simulink library "Lib_EMTAT"  (R2023b)
settings: Solver=VariableStepAuto  StartTime=0.0  StopTime=10.0  RelTol=1e-3
undefined symbols (not defined in the file): MWS
libraries: simulink x34
(part 2 of 4)

== system Lib_EMTAT/Components/Power Flow/Cable ==
  note: Memory block used to break algebraic loop.
  "V_1, V" : Inport
  "I, A" : Inport  Port=2
  Fail? : Inport  Port=3
  "I(t-1), A" : Inport  Port=4
  Bus Creator : BusCreator  Inputs=7
  Constant : Constant  Value=R
  Divide{,1..3} (4 alike) : Product  Inputs=**
  Failure Determination : Subsystem
  Fix Zero Voltage Problem : Subsystem
  Open Circuit Failure - Current : Subsystem
  Open Circuit Failure - Voltage : Subsystem
  Square : Math  Operator=square
  Sum : Sum  Inputs=|-+
  "V_2, V" : Outport
  Outputs : Outport  Port=2
  "Ploss, W" : Outport  Port=3
  "I, A " : Outport  Port=4
  "I(t), A" : Outport  Port=5
  wires:
  [OCFail] -> Open Circuit Failure - Voltage/1(Failed?)
  Fix Zero Voltage Problem/1(Vout) -> Open Circuit Failure - Voltage/2(Vout)
  [OCFail] -> Open Circuit Failure - Current/1(Failed?)
  Open Circuit Failure - Current/1("Iin/Iout ") -> "I, A "/1, [Iin], Divide2/2, Divide3/1, Square/1
  "I, A"/1 -> "I(t), A"/1, Open Circuit Failure - Current/2(Iin/Iout)
  Fail?/1 -> Failure Determination/1(Fail?)
  Failure Determination/1(OCFail) -> [OCFail]
  "I(t-1), A"/1 -> Divide/1
  Divide/1 -> Sum/1
  "V_1, V"/1 -> Divide2/1, Sum/2, Fix Zero Voltage Problem/2(Vin), [Vin]
  Sum/1 -> Fix Zero Voltage Problem/1("Vout "), Divide3/2
  [Iin] -> Bus Creator/3  "I; A"
  [Vout] -> Bus Creator/5  "V_2; V"
  [Vin] -> Bus Creator/4  "V_1; V"
  Bus Creator/1 -> Outputs/1
  [R] -> Bus Creator/6  "R; ohm"
  Constant/1 -> Divide1/2, [R], Divide/2
  Square/1 -> Divide1/1
  Divide1/1 -> [Ploss], "Ploss, W"/1
  [Pin] -> Bus Creator/2  "P_1; W"
  [Pout] -> Bus Creator/1  "P_2; W"
  Divide2/1 -> [Pin]
  Divide3/1 -> [Pout]
  [Ploss] -> Bus Creator/7  "Ploss; W"
  Open Circuit Failure - Voltage/1("Vout ") -> "V_2, V"/1, [Vout]

== system Lib_EMTAT/Components/Power Flow/Current Distribution ==
  "I, A" : Inport
  "Idmd, A" : Inport  Port=2
  MATLAB Function : MATLAB Function  TreatAsAtomicUnit=on
  "Isplit, A" : Outport
  wires:
  "Idmd, A"/1 -> MATLAB Function/2(Idmd)
  MATLAB Function/1(Isplit) -> "Isplit, A"/1
  "I, A"/1 -> MATLAB Function/1(I)

== system Lib_EMTAT/Components/Power Flow/Current Junction ==
  I : Inport
  MATLAB Function : MATLAB Function  TreatAsAtomicUnit=on
  Isum : Outport
  wires:
  I/1 -> MATLAB Function/1(u)
  MATLAB Function/1(y) -> Isum/1

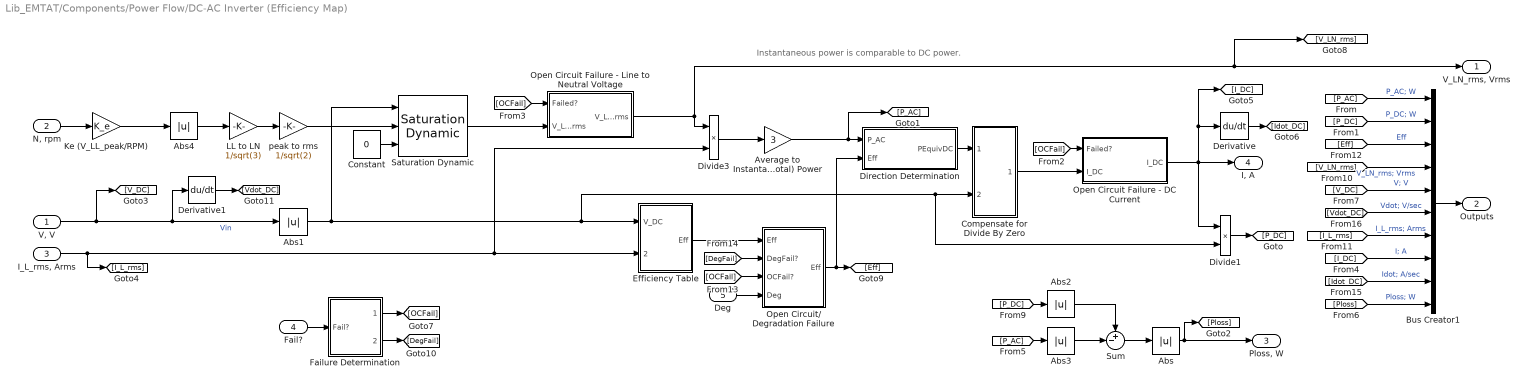
== system Lib_EMTAT/Components/Power Flow/DC-AC Inverter (Efficiency Map) ==
  note: Instantaneous power is comparable to DC power.
  "V, V" : Inport
  "N, rpm" : Inport  Port=2
  "I_L_rms, Arms" : Inport  Port=3
  Fail? : Inport  Port=4
  Deg : Inport  Port=5
  Abs{,1..4} (5 alike) : Abs  SaturateOnIntegerOverflow=off
  Average to Instantaneous (Total) Power : Gain  Gain=3
  Bus Creator1 : BusCreator  Inputs=10
  Compensate for Divide By Zero : Subsystem
  Constant : Constant  Value=0
  Derivative : Derivative
  Derivative1 : Derivative
  Direction Determination : Subsystem
  Divide1 : Product  Inputs=**
  Divide3 : Product  Inputs=**
  Efficiency Table : Subsystem
  Failure Determination : Subsystem
  Ke (V_LL_peak/RPM) : Gain  Gain=K_e
  LL to LN : Gain  Gain=1/sqrt(3)
  Open Circuit Failure - DC Current : Subsystem
  Open Circuit Failure - Line to Neutral Voltage : Subsystem
  Open Circuit/ Degradation Failure : Subsystem
  Saturation Dynamic : simulink/Discontinuities/Saturation Dynamic  OutMin=[]  OutMax=[]  OutDataTypeStr=Inherit: Same as second input  OutDataType=fixdt(1, 16)  OutScaling=2^-10  DoSatur=off
  Sum : Sum  Inputs=+-|
  peak to rms : Gain  Gain=1/sqrt(2)
  "V_LN_rms, Vrms" : Outport
  Outputs : Outport  Port=2
  "Ploss, W" : Outport  Port=3
  "I, A" : Outport  Port=4
  wires:
  peak to rms/1 -> Saturation Dynamic/2
  Constant/1 -> Saturation Dynamic/3
  Divide3/1 -> Average to Instantaneous (Total) Power/1
  Abs4/1 -> LL to LN/1
  Abs1/1 -> Efficiency Table/1(V_DC), Compensate for Divide By Zero/2(V_DC), Divide1/2, Saturation Dynamic/1
  Divide1/1 -> [P_DC]
  Direction Determination/1(PEquivDC) -> Compensate for Divide By Zero/1(PEquivDC)
  Bus Creator1/1 -> Outputs/1
  [P_AC] -> Bus Creator1/1  "P_AC; W"
  [P_DC] -> Bus Creator1/2  "P_DC; W"
  "N, rpm"/1 -> Ke (V_LL_peak/RPM)/1
  Open Circuit/ Degradation Failure/1("Eff ") -> [Eff], Direction Determination/2(Eff)
  Open Circuit Failure - DC Current/1("I_DC ") -> Divide1/1, "I, A"/1, Derivative/1, [I_DC]
  Average to Instantaneous (Total) Power/1 -> Direction Determination/1(P_AC), [P_AC]
  "V, V"/1 -> Derivative1/1, Abs1/1, [V_DC]  "Vin"
  Ke (V_LL_peak/RPM)/1 -> Abs4/1
  "I_L_rms, Arms"/1 -> Efficiency Table/2(I_L_rms), Divide3/2, [I_L_rms]
  [V_LN_rms] -> Bus Creator1/4  "V_LN_rms; Vrms"
  [V_DC] -> Bus Creator1/5  "V; V"
  [I_DC] -> Bus Creator1/8  "I; A"
  [Ploss] -> Bus Creator1/10  "Ploss; W"
  [I_L_rms] -> Bus Creator1/7  "I_L_rms; Arms"
  [Eff] -> Bus Creator1/3  "Eff"
  LL to LN/1 -> peak to rms/1
  Compensate for Divide By Zero/1(I_DC) -> Open Circuit Failure - DC Current/2(I_DC)
  [OCFail] -> Open Circuit Failure - DC Current/1(Failed?)
  Saturation Dynamic/1 -> Open Circuit Failure - Line to Neutral Voltage/2(V_LN_rms)
  [OCFail] -> Open Circuit Failure - Line to Neutral Voltage/1(Failed?)
  Open Circuit Failure - Line to Neutral Voltage/1("V_LN_rms ") -> [V_LN_rms], "V_LN_rms, Vrms"/1, Divide3/1
  Efficiency Table/1(Eff) -> Open Circuit/ Degradation Failure/1(Eff)
  Failure Determination/2(DegFail) -> [DegFail]
  Failure Determination/1(OCFail) -> [OCFail]
  Fail?/1 -> Failure Determination/1(Fail?)
  Deg/1 -> Open Circuit/ Degradation Failure/4(Deg)
  [OCFail] -> Open Circuit/ Degradation Failure/3(OCFail?)
  [DegFail] -> Open Circuit/ Degradation Failure/2(DegFail?)
  Derivative/1 -> [Idot_DC]
  Derivative1/1 -> [Vdot_DC]
  [Idot_DC] -> Bus Creator1/9  "Idot; A/sec"
  [Vdot_DC] -> Bus Creator1/6  "Vdot; V/sec"
  Sum/1 -> Abs/1
  [P_DC] -> Abs2/1
  Abs3/1 -> Sum/2
  [P_AC] -> Abs3/1
  Abs2/1 -> Sum/1
  Abs/1 -> [Ploss], "Ploss, W"/1

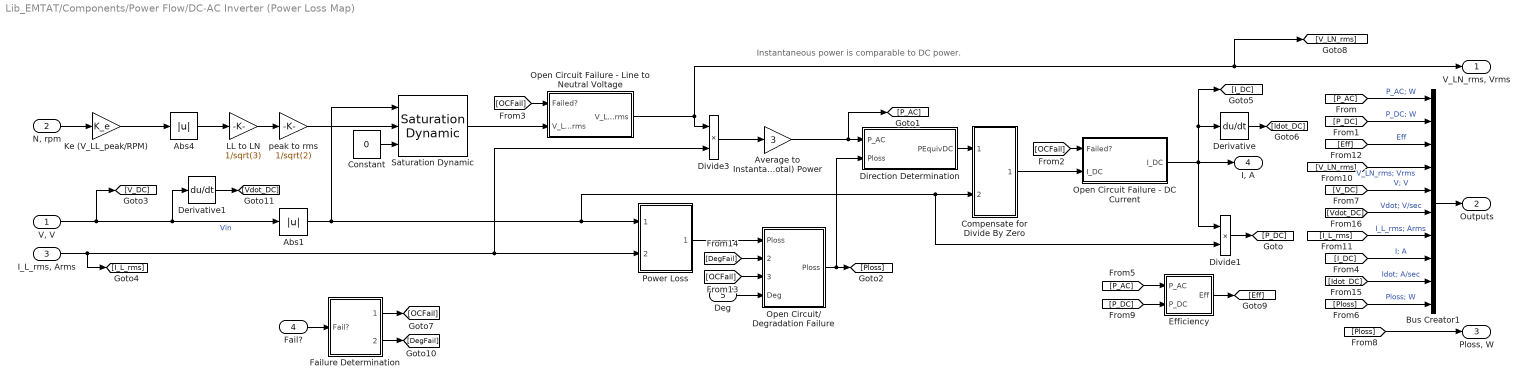
== system Lib_EMTAT/Components/Power Flow/DC-AC Inverter (Power Loss Map) ==
  note: Instantaneous power is comparable to DC power.
  "V, V" : Inport
  "N, rpm" : Inport  Port=2
  "I_L_rms, Arms" : Inport  Port=3
  Fail? : Inport  Port=4
  Deg : Inport  Port=5
  Abs1 : Abs  SaturateOnIntegerOverflow=off
  Abs4 : Abs  SaturateOnIntegerOverflow=off
  Average to Instantaneous (Total) Power : Gain  Gain=3
  Bus Creator1 : BusCreator  Inputs=10
  Compensate for Divide By Zero : Subsystem
  Constant : Constant  Value=0
  Derivative : Derivative
  Derivative1 : Derivative
  Direction Determination : Subsystem
  Divide1 : Product  Inputs=**
  Divide3 : Product  Inputs=**
  Efficiency : Subsystem
  Failure Determination : Subsystem
  Ke (V_LL_peak/RPM) : Gain  Gain=K_e
  LL to LN : Gain  Gain=1/sqrt(3)
  Open Circuit Failure - DC Current : Subsystem
  Open Circuit Failure - Line to Neutral Voltage : Subsystem
  Open Circuit/ Degradation Failure : Subsystem
  Power Loss : Subsystem
  Saturation Dynamic : simulink/Discontinuities/Saturation Dynamic  OutMin=[]  OutMax=[]  OutDataTypeStr=Inherit: Same as second input  OutDataType=fixdt(1, 16)  OutScaling=2^-10  DoSatur=off
  peak to rms : Gain  Gain=1/sqrt(2)
  "V_LN_rms, Vrms" : Outport
  Outputs : Outport  Port=2
  "Ploss, W" : Outport  Port=3
  "I, A" : Outport  Port=4
  wires:
  [Vdot_DC] -> Bus Creator1/6  "Vdot; V/sec"
  [Idot_DC] -> Bus Creator1/9  "Idot; A/sec"
  Derivative1/1 -> [Vdot_DC]
  Derivative/1 -> [Idot_DC]
  [DegFail] -> Open Circuit/ Degradation Failure/2(DegFail?)
  [OCFail] -> Open Circuit/ Degradation Failure/3(OCFail?)
  Deg/1 -> Open Circuit/ Degradation Failure/4(Deg)
  Fail?/1 -> Failure Determination/1(Fail?)
  Failure Determination/1(OCFail) -> [OCFail]
  Failure Determination/2(DegFail) -> [DegFail]
  Power Loss/1(Ploss) -> Open Circuit/ Degradation Failure/1(Ploss)
  Open Circuit Failure - Line to Neutral Voltage/1("V_LN_rms ") -> Divide3/1, "V_LN_rms, Vrms"/1, [V_LN_rms]
  [OCFail] -> Open Circuit Failure - Line to Neutral Voltage/1(Failed?)
  Saturation Dynamic/1 -> Open Circuit Failure - Line to Neutral Voltage/2(V_LN_rms)
  [OCFail] -> Open Circuit Failure - DC Current/1(Failed?)
  Compensate for Divide By Zero/1(I_DC) -> Open Circuit Failure - DC Current/2(I_DC)
  LL to LN/1 -> peak to rms/1
  [Eff] -> Bus Creator1/3  "Eff"
  Efficiency/1(Eff) -> [Eff]
  [P_AC] -> Efficiency/1(P_AC)
  [P_DC] -> Efficiency/2(P_DC)
  [I_L_rms] -> Bus Creator1/7  "I_L_rms; Arms"
  [Ploss] -> Bus Creator1/10  "Ploss; W"
  [I_DC] -> Bus Creator1/8  "I; A"
  [V_DC] -> Bus Creator1/5  "V; V"
  [V_LN_rms] -> Bus Creator1/4  "V_LN_rms; Vrms"
  "I_L_rms, Arms"/1 -> [I_L_rms], Divide3/2, Power Loss/2(I_L_rms)
  [Ploss] -> "Ploss, W"/1
  Ke (V_LL_peak/RPM)/1 -> Abs4/1
  "V, V"/1 -> [V_DC], Abs1/1, Derivative1/1  "Vin"
  Average to Instantaneous (Total) Power/1 -> [P_AC], Direction Determination/1(P_AC)
  Open Circuit Failure - DC Current/1("I_DC ") -> [I_DC], Derivative/1, "I, A"/1, Divide1/1
  Open Circuit/ Degradation Failure/1("Ploss ") -> [Ploss], Direction Determination/2(Ploss)
  "N, rpm"/1 -> Ke (V_LL_peak/RPM)/1
  [P_DC] -> Bus Creator1/2  "P_DC; W"
  [P_AC] -> Bus Creator1/1  "P_AC; W"
  Bus Creator1/1 -> Outputs/1
  Direction Determination/1(PEquivDC) -> Compensate for Divide By Zero/1(PEquivDC)
  Divide1/1 -> [P_DC]
  Abs1/1 -> Saturation Dynamic/1, Divide1/2, Compensate for Divide By Zero/2(V_DC), Power Loss/1(V_DC)
  Abs4/1 -> LL to LN/1
  Divide3/1 -> Average to Instantaneous (Total) Power/1
  Constant/1 -> Saturation Dynamic/3
  peak to rms/1 -> Saturation Dynamic/2

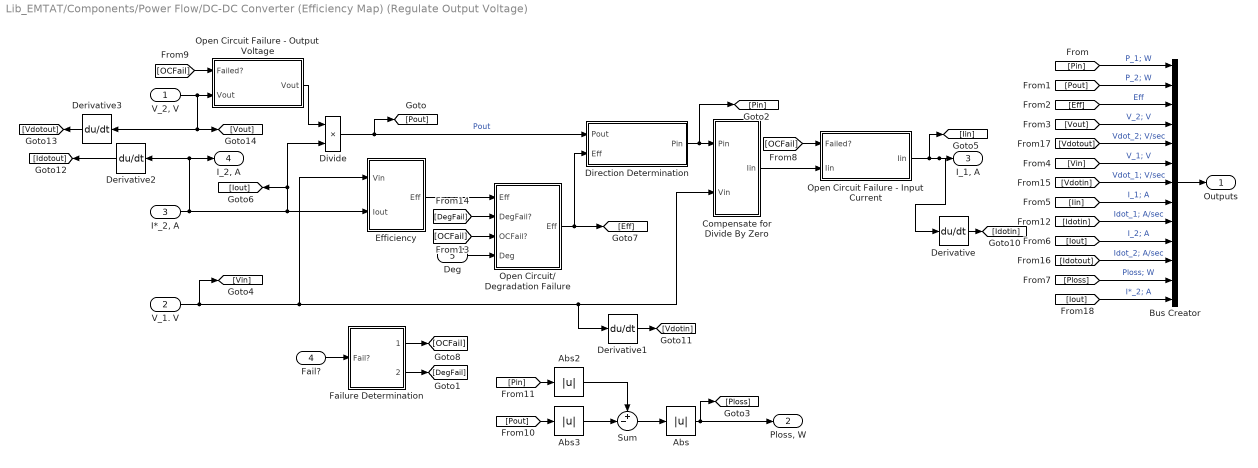
== system Lib_EMTAT/Components/Power Flow/DC-DC Converter (Efficiency Map) (Regulate Output Voltage) ==
  "V_2, V" : Inport
  V_1. V : Inport  Port=2
  "I*_2, A" : Inport  Port=3
  Fail? : Inport  Port=4
  Deg : Inport  Port=5
  Abs : Abs  SaturateOnIntegerOverflow=off
  Abs2 : Abs  SaturateOnIntegerOverflow=off
  Abs3 : Abs  SaturateOnIntegerOverflow=off
  Bus Creator : BusCreator  Inputs=13
  Compensate for Divide By Zero : Subsystem
  Derivative{,1..3} (4 alike) : Derivative
  Direction Determination : Subsystem
  Divide : Product  Inputs=**
  Efficiency : Subsystem
  Failure Determination : Subsystem
  Open Circuit Failure - Input Current : Subsystem
  Open Circuit Failure - Output Voltage : Subsystem
  Open Circuit/ Degradation Failure : Subsystem
  Sum : Sum  Inputs=+-|
  Outputs : Outport
  "Ploss, W" : Outport  Port=2
  "I_1, A" : Outport  Port=3
  "I_2, A" : Outport  Port=4
  wires:
  [Iout] -> Bus Creator/13  "I*_2; A"
  Fail?/1 -> Failure Determination/1(Fail?)
  Failure Determination/1(OCFail) -> [OCFail]
  Failure Determination/2(DegFail) -> [DegFail]
  Efficiency/1(Eff) -> Open Circuit/ Degradation Failure/1(Eff)
  Deg/1 -> Open Circuit/ Degradation Failure/4(Deg)
  [DegFail] -> Open Circuit/ Degradation Failure/2(DegFail?)
  [OCFail] -> Open Circuit/ Degradation Failure/3(OCFail?)
  [OCFail] -> Open Circuit Failure - Output Voltage/1(Failed?)
  Open Circuit Failure - Output Voltage/1("Vout   ") -> Divide/1
  [OCFail] -> Open Circuit Failure - Input Current/1(Failed?)
  Compensate for Divide By Zero/1(Iin) -> Open Circuit Failure - Input Current/2(Iin)
  "V_2, V"/1 -> Open Circuit Failure - Output Voltage/2(Vout), [Vout], Derivative3/1
  V_1. V/1 -> [Vin], Derivative1/1, Compensate for Divide By Zero/2(Vin), Efficiency/1(Vin)
  Open Circuit Failure - Input Current/1("Iin  ") -> Derivative/1, "I_1, A"/1, [Iin]
  Open Circuit/ Degradation Failure/1("Eff ") -> Direction Determination/2(Eff), [Eff]
  Divide/1 -> Direction Determination/1(Pout), [Pout]  "Pout"
  Bus Creator/1 -> Outputs/1
  Direction Determination/1(Pin) -> [Pin], Compensate for Divide By Zero/1(Pin)
  [Pin] -> Bus Creator/1  "P_1; W"
  [Pout] -> Bus Creator/2  "P_2; W"
  [Eff] -> Bus Creator/3  "Eff"
  [Vout] -> Bus Creator/4  "V_2; V"
  [Vin] -> Bus Creator/6  "V_1; V"
  [Iin] -> Bus Creator/8  "I_1; A"
  "I*_2, A"/1 -> "I_2, A"/1, Derivative2/1, Efficiency/2(Iout), [Iout], Divide/2
  [Iout] -> Bus Creator/10  "I_2; A"
  [Ploss] -> Bus Creator/12  "Ploss; W"
  Derivative/1 -> [Idotin]
  Derivative1/1 -> [Vdotin]
  Derivative2/1 -> [Idotout]
  Derivative3/1 -> [Vdotout]
  [Idotout] -> Bus Creator/11  "Idot_2; A/sec"
  [Idotin] -> Bus Creator/9  "Idot_1; A/sec"
  [Vdotin] -> Bus Creator/7  "Vdot_1; V/sec"
  [Vdotout] -> Bus Creator/5  "Vdot_2; V/sec"
  [Pout] -> Abs3/1
  Abs3/1 -> Sum/2
  [Pin] -> Abs2/1
  Sum/1 -> Abs/1
  Abs2/1 -> Sum/1
  Abs/1 -> "Ploss, W"/1, [Ploss]

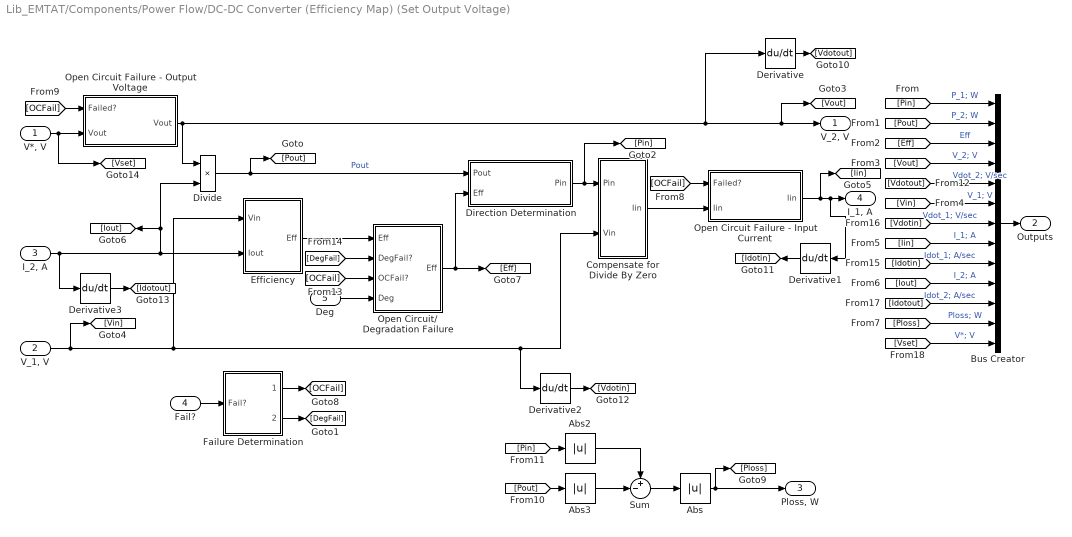
== system Lib_EMTAT/Components/Power Flow/DC-DC Converter (Efficiency Map) (Set Output Voltage) ==
  "V*, V" : Inport
  "V_1, V" : Inport  Port=2
  "I_2, A" : Inport  Port=3
  Fail? : Inport  Port=4
  Deg : Inport  Port=5
  Abs : Abs  SaturateOnIntegerOverflow=off
  Abs2 : Abs  SaturateOnIntegerOverflow=off
  Abs3 : Abs  SaturateOnIntegerOverflow=off
  Bus Creator : BusCreator  Inputs=13
  Compensate for Divide By Zero : Subsystem
  Derivative{,1..3} (4 alike) : Derivative
  Direction Determination : Subsystem
  Divide : Product  Inputs=**
  Efficiency : Subsystem
  Failure Determination : Subsystem
  Open Circuit Failure - Input Current : Subsystem
  Open Circuit Failure - Output Voltage : Subsystem
  Open Circuit/ Degradation Failure : Subsystem
  Sum : Sum  Inputs=+-|
  "V_2, V" : Outport
  Outputs : Outport  Port=2
  "Ploss, W" : Outport  Port=3
  "I_1, A" : Outport  Port=4
  wires:
  [Ploss] -> Bus Creator/12  "Ploss; W"
  [Iout] -> Bus Creator/10  "I_2; A"
  "I_2, A"/1 -> Derivative3/1, Divide/2, [Iout], Efficiency/2(Iout)
  [Iin] -> Bus Creator/8  "I_1; A"
  [Vin] -> Bus Creator/6  "V_1; V"
  [Vout] -> Bus Creator/4  "V_2; V"
  [Eff] -> Bus Creator/3  "Eff"
  [Pout] -> Bus Creator/2  "P_2; W"
  [Pin] -> Bus Creator/1  "P_1; W"
  Direction Determination/1(Pin) -> Compensate for Divide By Zero/1(Pin), [Pin]
  Bus Creator/1 -> Outputs/1
  Divide/1 -> Direction Determination/1(Pout), [Pout]  "Pout"
  Open Circuit/ Degradation Failure/1("Eff ") -> Direction Determination/2(Eff), [Eff]
  Open Circuit Failure - Input Current/1("Iin  ") -> Derivative1/1, "I_1, A"/1, [Iin]
  "V_1, V"/1 -> Efficiency/1(Vin), Derivative2/1, Compensate for Divide By Zero/2(Vin), [Vin]
  "V*, V"/1 -> [Vset], Open Circuit Failure - Output Voltage/2(Vout)
  Compensate for Divide By Zero/1(Iin) -> Open Circuit Failure - Input Current/2(Iin)
  [OCFail] -> Open Circuit Failure - Input Current/1(Failed?)
  Open Circuit Failure - Output Voltage/1("Vout   ") -> Derivative/1, [Vout], "V_2, V"/1, Divide/1
  [OCFail] -> Open Circuit Failure - Output Voltage/1(Failed?)
  [OCFail] -> Open Circuit/ Degradation Failure/3(OCFail?)
  [DegFail] -> Open Circuit/ Degradation Failure/2(DegFail?)
  Deg/1 -> Open Circuit/ Degradation Failure/4(Deg)
  Efficiency/1(Eff) -> Open Circuit/ Degradation Failure/1(Eff)
  Failure Determination/2(DegFail) -> [DegFail]
  Failure Determination/1(OCFail) -> [OCFail]
  Fail?/1 -> Failure Determination/1(Fail?)
  Derivative/1 -> [Vdotout]
  Derivative1/1 -> [Idotin]
  Derivative2/1 -> [Vdotin]
  Derivative3/1 -> [Idotout]
  [Idotout] -> Bus Creator/11  "Idot_2; A/sec"
  [Idotin] -> Bus Creator/9  "Idot_1; A/sec"
  [Vdotin] -> Bus Creator/7  "Vdot_1; V/sec"
  [Vdotout] -> Bus Creator/5  "Vdot_2; V/sec"
  [Vset] -> Bus Creator/13  "V*; V"
  Abs/1 -> "Ploss, W"/1, [Ploss]
  Abs3/1 -> Sum/2
  [Pout] -> Abs3/1
  Sum/1 -> Abs/1
  Abs2/1 -> Sum/1
  [Pin] -> Abs2/1

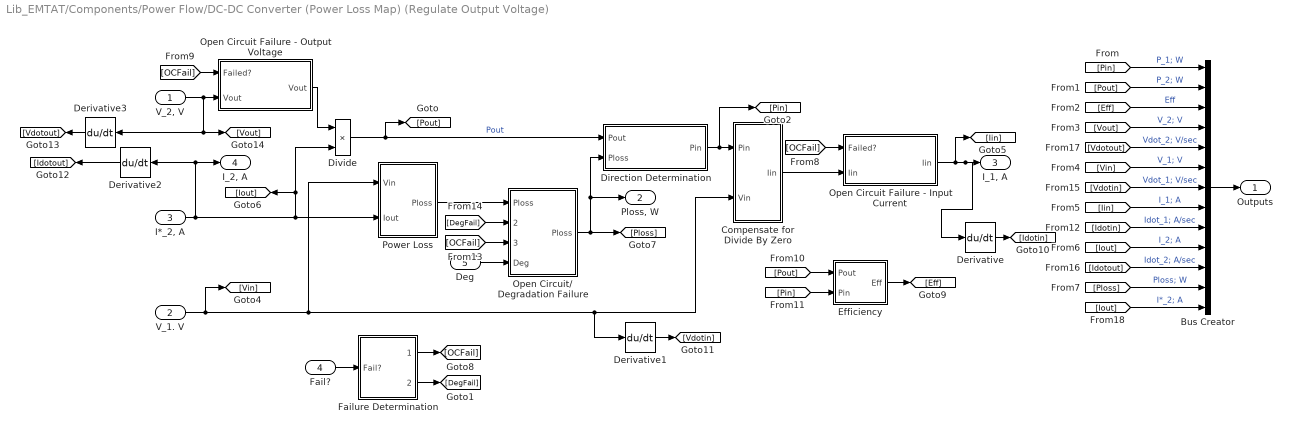
== system Lib_EMTAT/Components/Power Flow/DC-DC Converter (Power Loss Map) (Regulate Output Voltage) ==
  "V_2, V" : Inport
  V_1. V : Inport  Port=2
  "I*_2, A" : Inport  Port=3
  Fail? : Inport  Port=4
  Deg : Inport  Port=5
  Bus Creator : BusCreator  Inputs=13
  Compensate for Divide By Zero : Subsystem
  Derivative{,1..3} (4 alike) : Derivative
  Direction Determination : Subsystem
  Divide : Product  Inputs=**
  Efficiency : Subsystem
  Failure Determination : Subsystem
  Open Circuit Failure - Input Current : Subsystem
  Open Circuit Failure - Output Voltage : Subsystem
  Open Circuit/ Degradation Failure : Subsystem
  Power Loss : Subsystem
  Outputs : Outport
  "Ploss, W" : Outport  Port=2
  "I_1, A" : Outport  Port=3
  "I_2, A" : Outport  Port=4
  wires:
  [Vdotout] -> Bus Creator/5  "Vdot_2; V/sec"
  [Vdotin] -> Bus Creator/7  "Vdot_1; V/sec"
  [Idotin] -> Bus Creator/9  "Idot_1; A/sec"
  [Idotout] -> Bus Creator/11  "Idot_2; A/sec"
  Derivative3/1 -> [Vdotout]
  Derivative2/1 -> [Idotout]
  Derivative1/1 -> [Vdotin]
  Derivative/1 -> [Idotin]
  [Ploss] -> Bus Creator/12  "Ploss; W"
  [Iout] -> Bus Creator/10  "I_2; A"
  "I*_2, A"/1 -> Divide/2, [Iout], Power Loss/2(Iout), Derivative2/1, "I_2, A"/1
  [Iin] -> Bus Creator/8  "I_1; A"
  [Vin] -> Bus Creator/6  "V_1; V"
  [Vout] -> Bus Creator/4  "V_2; V"
  [Eff] -> Bus Creator/3  "Eff"
  [Pout] -> Bus Creator/2  "P_2; W"
  [Pin] -> Bus Creator/1  "P_1; W"
  Direction Determination/1(Pin) -> Compensate for Divide By Zero/1(Pin), [Pin]
  Bus Creator/1 -> Outputs/1
  Divide/1 -> Direction Determination/1(Pout), [Pout]  "Pout"
  Open Circuit/ Degradation Failure/1("Ploss ") -> "Ploss, W"/1, Direction Determination/2(Ploss), [Ploss]
  Open Circuit Failure - Input Current/1("Iin  ") -> [Iin], "I_1, A"/1, Derivative/1
  V_1. V/1 -> Power Loss/1(Vin), Compensate for Divide By Zero/2(Vin), Derivative1/1, [Vin]
  "V_2, V"/1 -> Derivative3/1, [Vout], Open Circuit Failure - Output Voltage/2(Vout)
  [Pout] -> Efficiency/1(Pout)
  [Pin] -> Efficiency/2(Pin)
  Efficiency/1(Eff) -> [Eff]
  Compensate for Divide By Zero/1(Iin) -> Open Circuit Failure - Input Current/2(Iin)
  [OCFail] -> Open Circuit Failure - Input Current/1(Failed?)
  Open Circuit Failure - Output Voltage/1("Vout   ") -> Divide/1
  [OCFail] -> Open Circuit Failure - Output Voltage/1(Failed?)
  [OCFail] -> Open Circuit/ Degradation Failure/3(OCFail?)
  [DegFail] -> Open Circuit/ Degradation Failure/2(DegFail?)
  Deg/1 -> Open Circuit/ Degradation Failure/4(Deg)
  Power Loss/1(Ploss) -> Open Circuit/ Degradation Failure/1(Ploss)
  Failure Determination/2(DegFail) -> [DegFail]
  Failure Determination/1(OCFail) -> [OCFail]
  Fail?/1 -> Failure Determination/1(Fail?)
  [Iout] -> Bus Creator/13  "I*_2; A"

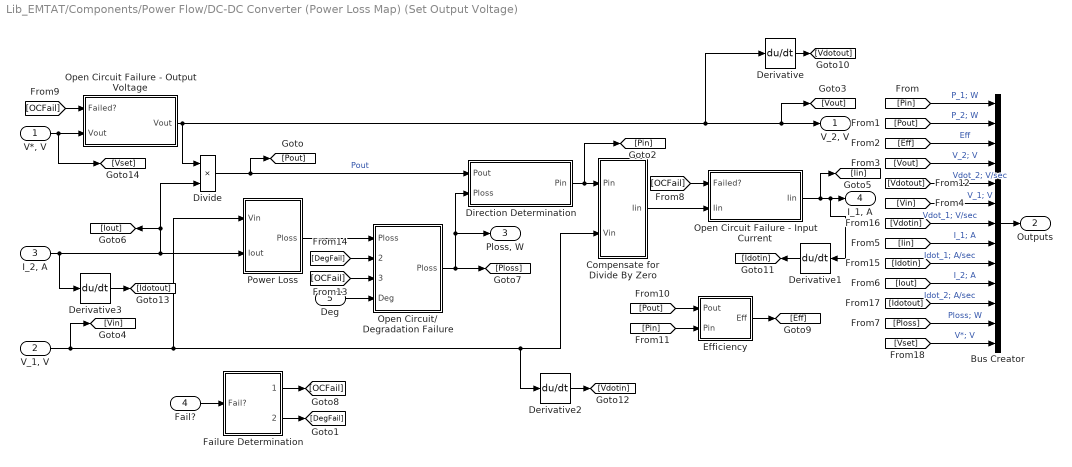
== system Lib_EMTAT/Components/Power Flow/DC-DC Converter (Power Loss Map) (Set Output Voltage) ==
  "V*, V" : Inport
  "V_1, V" : Inport  Port=2
  "I_2, A" : Inport  Port=3
  Fail? : Inport  Port=4
  Deg : Inport  Port=5
  Bus Creator : BusCreator  Inputs=13
  Compensate for Divide By Zero : Subsystem
  Derivative{,1..3} (4 alike) : Derivative
  Direction Determination : Subsystem
  Divide : Product  Inputs=**
  Efficiency : Subsystem
  Failure Determination : Subsystem
  Open Circuit Failure - Input Current : Subsystem
  Open Circuit Failure - Output Voltage : Subsystem
  Open Circuit/ Degradation Failure : Subsystem
  Power Loss : Subsystem
  "V_2, V" : Outport
  Outputs : Outport  Port=2
  "Ploss, W" : Outport  Port=3
  "I_1, A" : Outport  Port=4
  wires:
  [Vset] -> Bus Creator/13  "V*; V"
  [Vdotout] -> Bus Creator/5  "Vdot_2; V/sec"
  [Vdotin] -> Bus Creator/7  "Vdot_1; V/sec"
  [Idotin] -> Bus Creator/9  "Idot_1; A/sec"
  [Idotout] -> Bus Creator/11  "Idot_2; A/sec"
  Derivative3/1 -> [Idotout]
  Derivative2/1 -> [Vdotin]
  Derivative1/1 -> [Idotin]
  Derivative/1 -> [Vdotout]
  Fail?/1 -> Failure Determination/1(Fail?)
  Failure Determination/1(OCFail) -> [OCFail]
  Failure Determination/2(DegFail) -> [DegFail]
  Power Loss/1(Ploss) -> Open Circuit/ Degradation Failure/1(Ploss)
  Deg/1 -> Open Circuit/ Degradation Failure/4(Deg)
  [DegFail] -> Open Circuit/ Degradation Failure/2(DegFail?)
  [OCFail] -> Open Circuit/ Degradation Failure/3(OCFail?)
  [OCFail] -> Open Circuit Failure - Output Voltage/1(Failed?)
  Open Circuit Failure - Output Voltage/1("Vout   ") -> Divide/1, "V_2, V"/1, [Vout], Derivative/1
  [OCFail] -> Open Circuit Failure - Input Current/1(Failed?)
  Compensate for Divide By Zero/1(Iin) -> Open Circuit Failure - Input Current/2(Iin)
  Efficiency/1(Eff) -> [Eff]
  [Pin] -> Efficiency/2(Pin)
  [Pout] -> Efficiency/1(Pout)
  "V*, V"/1 -> Open Circuit Failure - Output Voltage/2(Vout), [Vset]
  "V_1, V"/1 -> [Vin], Compensate for Divide By Zero/2(Vin), Derivative2/1, Power Loss/1(Vin)
  Open Circuit Failure - Input Current/1("Iin  ") -> [Iin], "I_1, A"/1, Derivative1/1
  Open Circuit/ Degradation Failure/1("Ploss ") -> [Ploss], Direction Determination/2(Ploss), "Ploss, W"/1
  Divide/1 -> [Pout], Direction Determination/1(Pout)  "Pout"
  Bus Creator/1 -> Outputs/1
  Direction Determination/1(Pin) -> [Pin], Compensate for Divide By Zero/1(Pin)
  [Pin] -> Bus Creator/1  "P_1; W"
  [Pout] -> Bus Creator/2  "P_2; W"
  [Eff] -> Bus Creator/3  "Eff"
  [Vout] -> Bus Creator/4  "V_2; V"
  [Vin] -> Bus Creator/6  "V_1; V"
  [Iin] -> Bus Creator/8  "I_1; A"
  "I_2, A"/1 -> Power Loss/2(Iout), [Iout], Divide/2, Derivative3/1
  [Iout] -> Bus Creator/10  "I_2; A"
  [Ploss] -> Bus Creator/12  "Ploss; W"

== system Lib_EMTAT/Components/Power Flow/Electrical Bus ==
  "I, A" : Inport
  "V, V" : Inport  Port=2
  "Capacitance, F" : Constant  Value=C
  Divide : Product  Inputs=*/
  MATLAB Function : MATLAB Function  TreatAsAtomicUnit=on
  "V, V " : Outport
  "Vdot, V/sec" : Outport  Port=2
  wires:
  MATLAB Function/1(y) -> Divide/1
  "Capacitance, F"/1 -> Divide/2
  Divide/1 -> "Vdot, V/sec"/1
  "V, V"/1 -> "V, V "/1
  "I, A"/1 -> MATLAB Function/1(u)

== system Lib_EMTAT/Components/Power Flow/Mechanical Shaft ==
  note: Units
      | J : lb-ft-s^2
      | B : lb-ft-s
  "T, lbf-ft" : Inport
  Fail? : Inport  Port=2
  "N, rpm" : Inport  Port=3
  Abs : Abs  SaturateOnIntegerOverflow=off
  Bus Creator : BusCreator  Inputs=5
  Divide : Product  Inputs=*/
  Failure Determination : Subsystem
  Inertia (slug-ft^2 or lbf-ft-s^2) : Constant  Value=J
  RPM to rad/s : Gain  Gain=(2*pi)/60
  Shaft Break Failure : Subsystem
  Sum : Sum  Inputs=|+-
  "Viscous Damping Coefficient, lbf-ft-s" : Gain  Gain=B
  lbf-ft to Btu : Gain  Gain=0.00128507
  rad/s^2 to RPM/s : Gain  Gain=60/(2*pi)
  Outputs : Outport
  "Q, btu" : Outport  Port=2
  "Ndot, rpm/sec" : Outport  Port=3
  wires:
  Shaft Break Failure/1("T ") -> Sum/1
  [SBFail] -> Bus Creator/5  "SBFail"
  RPM to rad/s/1 -> "Viscous Damping Coefficient, lbf-ft-s"/1
  [SBFail] -> Shaft Break Failure/1(Failed?)
  Fail?/1 -> Failure Determination/1(Fail?)
  Failure Determination/1(SBFail) -> [SBFail]
  "N, rpm"/1 -> RPM to rad/s/1, [N]
  [Ndot] -> Bus Creator/3  "Ndot; rpm/sec"
  Inertia (slug-ft^2 or lbf-ft-s^2)/1 -> Divide/2
  Bus Creator/1 -> Outputs/1
  rad/s^2 to RPM/s/1 -> [Ndot], "Ndot, rpm/sec"/1
  Divide/1 -> rad/s^2 to RPM/s/1
  [Tnet] -> Bus Creator/1  "Tnet; lbf-ft"
  [N] -> Bus Creator/2  "N; rpm"
  [Heat] -> Bus Creator/4  "Heat; btu"
  Abs/1 -> "Q, btu"/1, [Heat]
  Sum/1 -> [Tnet], Divide/1
  "Viscous Damping Coefficient, lbf-ft-s"/1 -> Sum/2, lbf-ft to Btu/1
  lbf-ft to Btu/1 -> Abs/1
  "T, lbf-ft"/1 -> Shaft Break Failure/2(T)

== system Lib_EMTAT/Components/Power Flow/Power Supply (Set Voltage) ==
  "V*, V" : Inport
  "I, A" : Inport  Port=2
  Bus Creator : BusCreator  Inputs=3
  Divide : Product  Inputs=**
  MATLAB Function : MATLAB Function  TreatAsAtomicUnit=on
  Outputs : Outport
  "V, V" : Outport  Port=2
  wires:
  [Pdmd] -> Bus Creator/3  "P; W"
  [Idmdsum] -> Bus Creator/2  "Isum; A"
  [Vout] -> Bus Creator/1  "V; V"
  Divide/1 -> [Pdmd]
  Bus Creator/1 -> Outputs/1
  "V*, V"/1 -> "V, V"/1, Divide/1, [Vout]
  MATLAB Function/1(y) -> [Idmdsum], Divide/2  "Isum"
  "I, A"/1 -> MATLAB Function/1(u)

== system Lib_EMTAT/Components/Power Flow/Resistive Load Bank ==
  "V, V" : Inport
  "P*, W " : Inport  Port=2
  Fail? : Inport  Port=3
  Abs1 : Abs  SaturateOnIntegerOverflow=off
  Bus Creator : BusCreator  Inputs=5
  Divide2 : Product  Inputs=**
  Failure Determination : Subsystem
  Fix Divide By Zero. : Subsystem
  Fix Divide By Zero.1 : Subsystem
  Open Circuit Failure - Line to Neutral Voltage : Subsystem
  Square : Math  Operator=square
  Outputs : Outport
  "Ploss, W" : Outport  Port=2
  "I, A" : Outport  Port=3
  wires:
  Fix Divide By Zero.1/1(I) -> Open Circuit Failure - Line to Neutral Voltage/2(I)
  [OCFail] -> Open Circuit Failure - Line to Neutral Voltage/1(Failed?)
  Fail?/1 -> Failure Determination/1(Fail?)
  Failure Determination/1(OCFail) -> [OCFail]
  Abs1/1 -> Fix Divide By Zero./2(abs(Pset))
  Fix Divide By Zero./1(R) -> [R], Divide2/2
  Bus Creator/1 -> Outputs/1
  Square/1 -> Divide2/1, Fix Divide By Zero./1(I^2)
  "P*, W "/1 -> [Pset], Abs1/1, Fix Divide By Zero.1/2(Pset)  "Pset"
  "V, V"/1 -> [V], Fix Divide By Zero.1/1(V)  "V"
  Divide2/1 -> [Ploss], "Ploss, W"/1
  [V] -> Bus Creator/1  "V; V"
  [I] -> Bus Creator/2  "I; A"
  [Pset] -> Bus Creator/3  "P*; W"
  [R] -> Bus Creator/4  "R; ohm"
  [Ploss] -> Bus Creator/5  "Ploss; W"
  Open Circuit Failure - Line to Neutral Voltage/1("I ") -> Square/1, [I], "I, A"/1

== system Lib_EMTAT/Components/Power Flow/Supercapacitor ==
  note: Explanation for Convention Correction:
      | If Iout is positive, discharge the capacitor. This is because a positive current demand from a sink block means that the sink block needs current.
      | If Iout is negative, charge the capacitor. This is because a negative current demand from a sink block means that the sink block is giving current.
  "I, A " : Inport
  "V, V" : Inport  Port=2
  "I(t-1), A" : Inport  Port=3
  Bus Creator : BusCreator  Inputs=8
  Constant : Constant  Value=ESR
  Convention Correction : Gain  Gain=-1
  Discrete Derivative : simulink/Discrete/Discrete Derivative  gainval=1.0  ICPrevScaledInput=0.0  OutMin=[]  OutMax=[]  OutDataType=fixdt(1, 16)  OutScaling=2^-10  DoSatur=off
  Discrete Derivative1 : simulink/Discrete/Discrete Derivative  gainval=1.0  ICPrevScaledInput=0.0  OutMin=[]  OutMax=[]  OutDataType=fixdt(1, 16)  OutScaling=2^-10  DoSatur=off
  Discrete Derivative2 : simulink/Discrete/Discrete Derivative  gainval=1.0  ICPrevScaledInput=0.0  OutMin=[]  OutMax=[]  OutDataType=fixdt(1, 16)  OutScaling=2^-10  DoSatur=off
  Divide : Product  Inputs=**
  Divide1 : Product  Inputs=**
  Gain : Gain  Gain=1/C
  SOC : Subsystem
  Saturation : Saturate  UpperLimit=inf  LowerLimit=0
  Square1 : Math  Operator=square
  Sum : Sum  Inputs=|-+
  "Voltage, V to Energy, Wh" : Subsystem
  Warnings : Subsystem
  "Vout, V" : Outport
  Outputs : Outport  Port=2
  "Ploss, W" : Outport  Port=3
  "Vdot, V/sec" : Outport  Port=4
  "I(t), A" : Outport  Port=5
  wires:
  Saturation/1 -> "Voltage, V to Energy, Wh"/1(V), Discrete Derivative2/1, "Vout, V"/1, [Vout]
  "I(t-1), A"/1 -> Discrete Derivative1/1, Convention Correction/1, Divide/1
  "V, V"/1 -> Sum/2
  Divide/1 -> Sum/1
  Constant/1 -> Divide/2, Divide1/2
  Sum/1 -> Saturation/1
  [SOC] -> Warnings/1(SOC)
  [Vdotout] -> Bus Creator/5  "Vdot; V/sec"
  [SOCdot] -> Bus Creator/7  "SOCdot; %/sec"
  [Idotout] -> Bus Creator/3  "Idot; A/sec"
  Discrete Derivative/1 -> [SOCdot]
  Discrete Derivative2/1 -> [Vdotout]
  Discrete Derivative1/1 -> [Idotout]
  "Voltage, V to Energy, Wh"/1(E) -> [Energy], SOC/1(Energy (W-h))
  "I, A "/1 -> [Iout], "I(t), A"/1
  SOC/1(SOC) -> [SOC], Discrete Derivative/1
  [SOC] -> Bus Creator/6  "SOC; %"
  Divide1/1 -> [Ploss], "Ploss, W"/1
  [Ploss] -> Bus Creator/8  "Ploss; W"
  Square1/1 -> Divide1/1
  Bus Creator/1 -> Outputs/1
  [Vout] -> Bus Creator/4  "Vout; V"
  [Iout] -> Bus Creator/2  "I; A"
  [Energy] -> Bus Creator/1  "E; Wh"
  Gain/1 -> "Vdot, V/sec"/1  "Vdot"
  Convention Correction/1 -> Gain/1, Square1/1

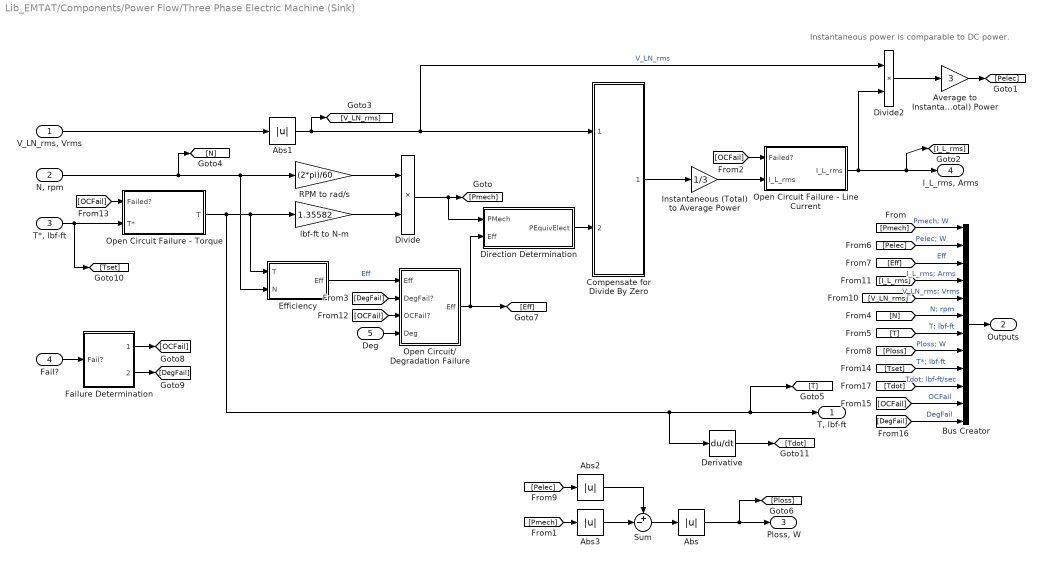
== system Lib_EMTAT/Components/Power Flow/Three Phase Electric Machine (Sink) ==
  note: Instantaneous power is comparable to DC power.
  "V_LN_rms, Vrms" : Inport
  "N, rpm" : Inport  Port=2
  "T*, lbf-ft" : Inport  Port=3
  Fail? : Inport  Port=4
  Deg : Inport  Port=5
  Abs{,1..3} (4 alike) : Abs  SaturateOnIntegerOverflow=off
  Average to Instantaneous (Total) Power : Gain  Gain=3
  Bus Creator : BusCreator  Inputs=12
  Compensate for Divide By Zero : Subsystem
  Derivative : Derivative
  Direction Determination : Subsystem
  Divide : Product  Inputs=**
  Divide2 : Product  Inputs=**
  Efficiency : Subsystem
  Failure Determination : Subsystem
  Instantaneous (Total) to Average Power : Gain  Gain=1/3
  Open Circuit Failure - Line Current : Subsystem
  Open Circuit Failure - Torque : Subsystem
  Open Circuit/ Degradation Failure : Subsystem
  RPM to rad/s : Gain  Gain=(2*pi)/60
  Sum : Sum  Inputs=+-|
  lbf-ft to N-m : Gain  Gain=1.35582
  "T, lbf-ft" : Outport
  Outputs : Outport  Port=2
  "Ploss, W" : Outport  Port=3
  "I_L_rms, Arms" : Outport  Port=4
  wires:
  [Tdot] -> Bus Creator/10  "Tdot; lbf-ft/sec"
  Derivative/1 -> [Tdot]
  [DegFail] -> Bus Creator/12  "DegFail"
  [OCFail] -> Bus Creator/11  "OCFail"
  [Tset] -> Bus Creator/9  "T*; lbf-ft"
  "T*, lbf-ft"/1 -> [Tset], Open Circuit Failure - Torque/2(T*)
  [OCFail] -> Open Circuit Failure - Torque/1(Failed?)
  [OCFail] -> Open Circuit/ Degradation Failure/3(OCFail?)
  Fail?/1 -> Failure Determination/1(Fail?)
  Deg/1 -> Open Circuit/ Degradation Failure/4(Deg)
  [DegFail] -> Open Circuit/ Degradation Failure/2(DegFail?)
  Open Circuit/ Degradation Failure/1("Eff ") -> [Eff], Direction Determination/2(Eff)
  Failure Determination/2(DegFail) -> [DegFail]
  Failure Determination/1(OCFail) -> [OCFail]
  [OCFail] -> Open Circuit Failure - Line Current/1(Failed?)
  Instantaneous (Total) to Average Power/1 -> Open Circuit Failure - Line Current/2(I_L_rms)
  Open Circuit Failure - Line Current/1("I_L_rms ") -> "I_L_rms, Arms"/1, [I_L_rms], Divide2/2
  Compensate for Divide By Zero/1(I_L_rms) -> Instantaneous (Total) to Average Power/1
  [N] -> Bus Creator/6  "N; rpm"
  [I_L_rms] -> Bus Creator/4  "I_L_rms; Arms"
  [V_LN_rms] -> Bus Creator/5  "V_LN_rms; Vrms"
  Abs1/1 -> [V_LN_rms], Divide2/1, Compensate for Divide By Zero/1(V_LN_rms)  "V_LN_rms"
  Abs3/1 -> Sum/2
  [Pmech] -> Abs3/1
  Abs2/1 -> Sum/1
  [Pelec] -> Abs2/1
  Bus Creator/1 -> Outputs/1
  Efficiency/1(Eff) -> Open Circuit/ Degradation Failure/1(Eff)  "Eff"
  "V_LN_rms, Vrms"/1 -> Abs1/1
  lbf-ft to N-m/1 -> Divide/2
  RPM to rad/s/1 -> Divide/1
  Open Circuit Failure - Torque/1("T  ") -> Efficiency/1(T), lbf-ft to N-m/1, "T, lbf-ft"/1, [T], Derivative/1
  Divide/1 -> [Pmech], Direction Determination/1(PMech)
  [Pmech] -> Bus Creator/1  "Pmech; W"
  Divide2/1 -> Average to Instantaneous (Total) Power/1
  [T] -> Bus Creator/7  "T; lbf-ft"
  [Eff] -> Bus Creator/3  "Eff"
  [Ploss] -> Bus Creator/8  "Ploss; W"
  Sum/1 -> Abs/1
  [Pelec] -> Bus Creator/2  "Pelec; W"
  Abs/1 -> [Ploss], "Ploss, W"/1
  Direction Determination/1(PEquivElect) -> Compensate for Divide By Zero/2(PEquivElect)
  "N, rpm"/1 -> Efficiency/2(N), RPM to rad/s/1, [N]
  Average to Instantaneous (Total) Power/1 -> [Pelec]

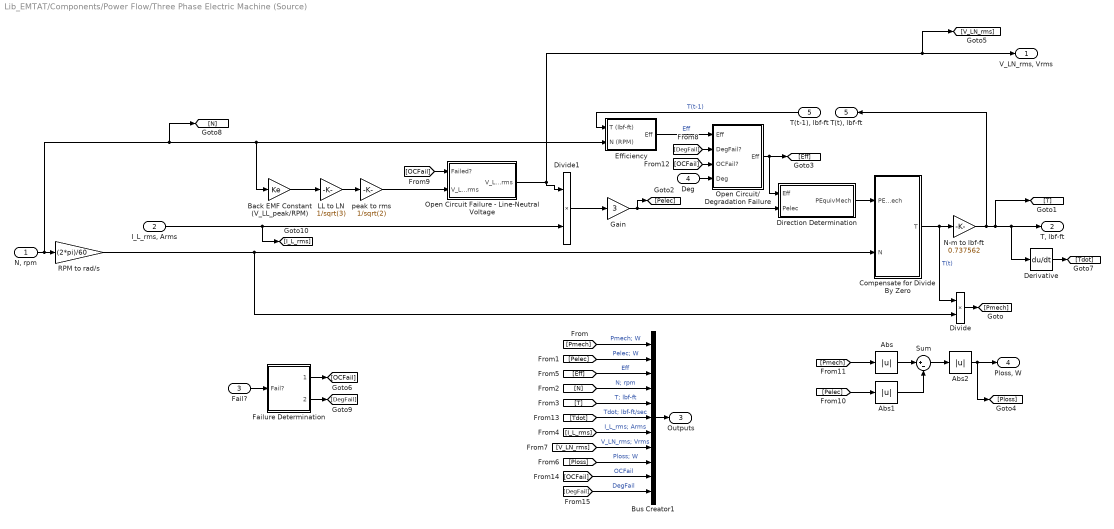
== system Lib_EMTAT/Components/Power Flow/Three Phase Electric Machine (Source) ==
  "N, rpm" : Inport
  "I_L_rms, Arms" : Inport  Port=2
  Fail? : Inport  Port=3
  Deg : Inport  Port=4
  "T(t-1), lbf-ft" : Inport  Port=5
  Abs : Abs  SaturateOnIntegerOverflow=off
  Abs1 : Abs  SaturateOnIntegerOverflow=off
  Abs2 : Abs  SaturateOnIntegerOverflow=off
  Back EMF Constant (V_LL_peak/RPM) : Gain  Gain=Ke
  Bus Creator1 : BusCreator  Inputs=11
  Compensate for Divide By Zero : Subsystem
  Derivative : Derivative
  Direction Determination : Subsystem
  Divide : Product  Inputs=**
  Divide1 : Product  Inputs=**
  Efficiency : Subsystem
  Failure Determination : Subsystem
  Gain : Gain  Gain=3
  LL to LN : Gain  Gain=1/sqrt(3)
  N-m to lbf-ft : Gain  Gain=0.737562
  Open Circuit Failure - Line-Neutral Voltage : Subsystem
  Open Circuit/ Degradation Failure : Subsystem
  RPM to rad/s : Gain  Gain=(2*pi)/60
  Sum : Sum  Inputs=|+-
  peak to rms : Gain  Gain=1/sqrt(2)
  "V_LN_rms, Vrms" : Outport
  "T, lbf-ft" : Outport  Port=2
  Outputs : Outport  Port=3
  "Ploss, W" : Outport  Port=4
  "T(t), lbf-ft" : Outport  Port=5
  wires:
  [DegFail] -> Bus Creator1/11  "DegFail"
  [OCFail] -> Bus Creator1/10  "OCFail"
  [Tdot] -> Bus Creator1/6  "Tdot; lbf-ft/sec"
  Derivative/1 -> [Tdot]
  peak to rms/1 -> Open Circuit Failure - Line-Neutral Voltage/2(V_LN_rms)
  Open Circuit Failure - Line-Neutral Voltage/1("V_LN_rms ") -> "V_LN_rms, Vrms"/1, [V_LN_rms], Divide1/1
  [OCFail] -> Open Circuit Failure - Line-Neutral Voltage/1(Failed?)
  Open Circuit/ Degradation Failure/1("Eff ") -> Direction Determination/1(Eff), [Eff]
  Deg/1 -> Open Circuit/ Degradation Failure/4(Deg)
  [DegFail] -> Open Circuit/ Degradation Failure/2(DegFail?)
  Efficiency/1(Eff) -> Open Circuit/ Degradation Failure/1(Eff)  "Eff"
  [OCFail] -> Open Circuit/ Degradation Failure/3(OCFail?)
  Failure Determination/1(OCFail) -> [OCFail]
  Failure Determination/2(DegFail) -> [DegFail]
  Fail?/1 -> Failure Determination/1(Fail?)
  N-m to lbf-ft/1 -> "T, lbf-ft"/1, Derivative/1, [T], "T(t), lbf-ft"/1
  Gain/1 -> Direction Determination/2(Pelec), [Pelec]
  LL to LN/1 -> peak to rms/1
  [Pmech] -> Abs/1
  [Pelec] -> Abs1/1
  Divide/1 -> [Pmech]
  Abs2/1 -> "Ploss, W"/1, [Ploss]
  Sum/1 -> Abs2/1
  Abs1/1 -> Sum/2
  Abs/1 -> Sum/1
  Bus Creator1/1 -> Outputs/1
  Direction Determination/1(PEquivMech) -> Compensate for Divide By Zero/1(PEquivMech)
  "T(t-1), lbf-ft"/1 -> Efficiency/1(T (lbf-ft))  "T(t-1)"
  Compensate for Divide By Zero/1(T) -> N-m to lbf-ft/1, Divide/1  "T(t)"
  Divide1/1 -> Gain/1
  Back EMF Constant (V_LL_peak/RPM)/1 -> LL to LN/1
  "N, rpm"/1 -> RPM to rad/s/1, Efficiency/2(N (RPM)), Back EMF Constant (V_LL_peak/RPM)/1, [N]
  [V_LN_rms] -> Bus Creator1/8  "V_LN_rms; Vrms"
  [I_L_rms] -> Bus Creator1/7  "I_L_rms; Arms"
  [Eff] -> Bus Creator1/3  "Eff"
  [T] -> Bus Creator1/5  "T; lbf-ft"
  [N] -> Bus Creator1/4  "N; rpm"
  [Pmech] -> Bus Creator1/1  "Pmech; W"
  [Ploss] -> Bus Creator1/9  "Ploss; W"
  [Pelec] -> Bus Creator1/2  "Pelec; W"
  RPM to rad/s/1 -> Divide/2, Compensate for Divide By Zero/2(N)
  "I_L_rms, Arms"/1 -> Divide1/2, [I_L_rms]

== system Lib_EMTAT/Components/Power Flow/AC-AC Transformer (Efficiency Map)/Compensate for Divide By Zero ==
  note: If Vin is not equal to zero, use its value.
      | If Vin is equal to zero, it will calculate a nan value for Iin. Set Iin to zero.
  P_AC_1 : Inport
  V_LN_rms_1 : Inport  Port=2
  Fix Divide By Zero. : Subsystem
  I_L_rms_1 : Outport
  wires:
  Fix Divide By Zero./1(I_L_rms_1) -> I_L_rms_1/1
  P_AC_1/1 -> Fix Divide By Zero./2(P_AC_1)
  V_LN_rms_1/1 -> Fix Divide By Zero./1(V_LN_rms_1)

== system Lib_EMTAT/Components/Power Flow/AC-AC Transformer (Efficiency Map)/Direction Determination ==
  P_AC_2 : Inport
  Eff : Inport  Port=2
  Divide : Product  Inputs=/*
  Divide1 : Product  Inputs=**
  Switch : Switch  Criteria=u2 > Threshold  SaturateOnIntegerOverflow=off  InputSameDT=off
  P_AC_1 : Outport
  wires:
  P_AC_2/1 -> Divide1/1, Divide/2, Switch/2
  Divide/1 -> Switch/1
  Divide1/1 -> Switch/3
  Eff/1 -> Divide/1, Divide1/2
  Switch/1 -> P_AC_1/1

== system Lib_EMTAT/Components/Power Flow/AC-AC Transformer (Efficiency Map)/Efficiency ==
  V_LN_rms_1 : Inport
  I_L_rms_2 : Inport  Port=2
  2-D Lookup Table : Lookup_n-D  BreakpointsForDimension1=X_C_VoltageAC1Vec_M  BreakpointsForDimension2=Y_C_CurrentAC2Vec_M  Table=T_C_EffArray_M  ExtrapMethod=Clip  UseLastTableValue=on  InternalRulePriority=Speed  RndMeth=Simplest
      settings: InputPortMap=u0,u1
  Abs : Abs  SaturateOnIntegerOverflow=off
  Abs1 : Abs  SaturateOnIntegerOverflow=off
  Eff : Outport
  wires:
  2-D Lookup Table/1 -> Eff/1
  I_L_rms_2/1 -> Abs1/1
  Abs1/1 -> 2-D Lookup Table/2
  Abs/1 -> 2-D Lookup Table/1
  V_LN_rms_1/1 -> Abs/1

== system Lib_EMTAT/Components/Power Flow/AC-AC Transformer (Efficiency Map)/Failure Determination ==
  Fail? : Inport
  Compare To Constant : simulink/Logic and Bit Operations/Compare To Constant  relop===  const=1  OutDataTypeStr=boolean
  Compare To Constant1 : simulink/Logic and Bit Operations/Compare To Constant  relop===  const=2  OutDataTypeStr=boolean
  Data Type Conversion : DataTypeConversion  OutDataTypeStr=double  SaturateOnIntegerOverflow=off  RndMeth=Floor
  Data Type Conversion1 : DataTypeConversion  OutDataTypeStr=double  SaturateOnIntegerOverflow=off  RndMeth=Floor
  Failure Mode : Constant  Value=FM
  Logical Operator : Logic  AllPortsSameDT=off  OutDataTypeStr=boolean
  Logical Operator1 : Logic  AllPortsSameDT=off  OutDataTypeStr=boolean
  OCFail : Outport
  DegFail : Outport  Port=2
  wires:
  Data Type Conversion/1 -> OCFail/1
  Data Type Conversion1/1 -> DegFail/1
  Fail?/1 -> Logical Operator/2, Logical Operator1/2
  Logical Operator1/1 -> Data Type Conversion1/1
  Compare To Constant1/1 -> Logical Operator1/1
  Logical Operator/1 -> Data Type Conversion/1
  Compare To Constant/1 -> Logical Operator/1
  Failure Mode/1 -> Compare To Constant/1, Compare To Constant1/1

== system Lib_EMTAT/Components/Power Flow/AC-AC Transformer (Efficiency Map)/Open Circuit Failure - DC Current ==
  Failed? : Inport
  I_L_rms_1 : Inport  Port=2
  Constant : Constant  Value=0
  IsInf : RelationalOperator  Operator=isInf  OutDataTypeStr=boolean  RndMeth=Simplest  InputSameDT=off
  IsNaN : RelationalOperator  Operator=isNaN  OutDataTypeStr=boolean  RndMeth=Simplest  InputSameDT=off
  Logical Operator : Logic  Operator=OR  Inputs=3  AllPortsSameDT=off  OutDataTypeStr=boolean
  Switch : Switch  Criteria=u2 > Threshold  SaturateOnIntegerOverflow=off  InputSameDT=off
  "I_L_rms_1 " : Outport
  wires:
  IsInf/1 -> Logical Operator/3
  IsNaN/1 -> Logical Operator/2
  Logical Operator/1 -> Switch/2
  Switch/1 -> "I_L_rms_1 "/1
  I_L_rms_1/1 -> Switch/3, IsInf/1, IsNaN/1
  Constant/1 -> Switch/1
  Failed?/1 -> Logical Operator/1

== system Lib_EMTAT/Components/Power Flow/AC-AC Transformer (Efficiency Map)/Open Circuit Failure - Line to Neutral Voltage ==
  Failed? : Inport
  V_LN_rms_2 : Inport  Port=2
  Constant : Constant  Value=0
  IsInf : RelationalOperator  Operator=isInf  OutDataTypeStr=boolean  RndMeth=Simplest  InputSameDT=off
  IsNaN : RelationalOperator  Operator=isNaN  OutDataTypeStr=boolean  RndMeth=Simplest  InputSameDT=off
  Logical Operator : Logic  Operator=OR  Inputs=3  AllPortsSameDT=off  OutDataTypeStr=boolean
  Switch : Switch  Criteria=u2 > Threshold  SaturateOnIntegerOverflow=off  InputSameDT=off
  "V_LN_rms_2 " : Outport
  wires:
  Failed?/1 -> Logical Operator/1
  Constant/1 -> Switch/1
  V_LN_rms_2/1 -> IsNaN/1, IsInf/1, Switch/3
  Switch/1 -> "V_LN_rms_2 "/1
  Logical Operator/1 -> Switch/2
  IsNaN/1 -> Logical Operator/2
  IsInf/1 -> Logical Operator/3

== system Lib_EMTAT/Components/Power Flow/AC-AC Transformer (Efficiency Map)/Open Circuit// Degradation Failure ==
  Eff : Inport
  DegFail? : Inport  Port=2
  OCFail? : Inport  Port=3
  Deg : Inport  Port=4
  Constant : Constant  Value=eps
  Constant1 : Constant
  Divide : Product  Inputs=**
  "If degradation failure, scale Eff." : Switch  Criteria=u2 > Threshold  SaturateOnIntegerOverflow=off  InputSameDT=off
  "If open circuit failure, set Eff = eps." : Switch  Criteria=u2 > Threshold  SaturateOnIntegerOverflow=off  InputSameDT=off
  Sum : Sum  Inputs=+-|
  "Eff " : Outport
  wires:
  DegFail?/1 -> "If degradation failure, scale Eff."/2
  "If degradation failure, scale Eff."/1 -> "If open circuit failure, set Eff = eps."/3
  Divide/1 -> "If degradation failure, scale Eff."/1
  "If open circuit failure, set Eff = eps."/1 -> "Eff "/1
  OCFail?/1 -> "If open circuit failure, set Eff = eps."/2
  Constant/1 -> "If open circuit failure, set Eff = eps."/1
  Sum/1 -> Divide/1
  Eff/1 -> "If degradation failure, scale Eff."/3, Divide/2
  Deg/1 -> Sum/2
  Constant1/1 -> Sum/1

== system Lib_EMTAT/Components/Power Flow/AC-AC Transformer (Power Loss Map)/Compensate for Divide By Zero ==
  note: If Vin is not equal to zero, use its value.
      | If Vin is equal to zero, it will calculate a nan value for Iin. Set Iin to zero.
  P_AC_1 : Inport
  V_LN_rms_1 : Inport  Port=2
  Fix Divide By Zero. : Subsystem
  I_L_rms_1 : Outport
  wires:
  V_LN_rms_1/1 -> Fix Divide By Zero./1(V_LN_rms_1)
  P_AC_1/1 -> Fix Divide By Zero./2(P_AC_1)
  Fix Divide By Zero./1(I_L_rms_1) -> I_L_rms_1/1

== system Lib_EMTAT/Components/Power Flow/AC-AC Transformer (Power Loss Map)/Direction Determination ==
  P_AC_2 : Inport
  Ploss : Inport  Port=2
  Add1 : Sum
  Switch : Switch  Criteria=u2 ~= 0  SaturateOnIntegerOverflow=off  InputSameDT=off
  P_AC_1 : Outport
  wires:
  Add1/1 -> Switch/1
  Switch/1 -> P_AC_1/1
  P_AC_2/1 -> Switch/2, Switch/3, Add1/2
  Ploss/1 -> Add1/1

== system Lib_EMTAT/Components/Power Flow/AC-AC Transformer (Power Loss Map)/Efficiency ==
  P_AC_2 : Inport
  P_AC_1 : Inport  Port=2
  Abs : Abs  SaturateOnIntegerOverflow=off
  Abs1 : Abs  SaturateOnIntegerOverflow=off
  Fix Divide By Zero. : Subsystem
  Fix Divide By Zero.1 : Subsystem
  GreaterThan : RelationalOperator  OutDataTypeStr=boolean  RndMeth=Simplest  InputSameDT=off
  Switch : Switch  Criteria=u2 > Threshold  SaturateOnIntegerOverflow=off  InputSameDT=off
  Eff : Outport
  wires:
  Switch/1 -> Eff/1
  GreaterThan/1 -> Switch/2
  Abs1/1 -> Fix Divide By Zero.1/2(abs(P_AC_2)), Fix Divide By Zero./1(abs(P_AC_2)), GreaterThan/2
  P_AC_1/1 -> Abs/1
  P_AC_2/1 -> Abs1/1
  Abs/1 -> Fix Divide By Zero.1/1(abs(P_AC_1)), Fix Divide By Zero./2(abs(P_AC_1)), GreaterThan/1
  Fix Divide By Zero./1(Eff) -> Switch/3
  Fix Divide By Zero.1/1(Eff) -> Switch/1

== system Lib_EMTAT/Components/Power Flow/AC-AC Transformer (Power Loss Map)/Failure Determination ==
  Fail? : Inport
  Compare To Constant : simulink/Logic and Bit Operations/Compare To Constant  relop===  const=1  OutDataTypeStr=boolean
  Compare To Constant1 : simulink/Logic and Bit Operations/Compare To Constant  relop===  const=2  OutDataTypeStr=boolean
  Data Type Conversion : DataTypeConversion  OutDataTypeStr=double  SaturateOnIntegerOverflow=off  RndMeth=Floor
  Data Type Conversion1 : DataTypeConversion  OutDataTypeStr=double  SaturateOnIntegerOverflow=off  RndMeth=Floor
  Failure Mode : Constant  Value=FM
  Logical Operator : Logic  AllPortsSameDT=off  OutDataTypeStr=boolean
  Logical Operator1 : Logic  AllPortsSameDT=off  OutDataTypeStr=boolean
  OCFail : Outport
  DegFail : Outport  Port=2
  wires:
  Failure Mode/1 -> Compare To Constant1/1, Compare To Constant/1
  Compare To Constant/1 -> Logical Operator/1
  Logical Operator/1 -> Data Type Conversion/1
  Compare To Constant1/1 -> Logical Operator1/1
  Logical Operator1/1 -> Data Type Conversion1/1
  Fail?/1 -> Logical Operator1/2, Logical Operator/2
  Data Type Conversion1/1 -> DegFail/1
  Data Type Conversion/1 -> OCFail/1

== system Lib_EMTAT/Components/Power Flow/AC-AC Transformer (Power Loss Map)/Open Circuit Failure - DC Current ==
  Failed? : Inport
  I_L_rms_1 : Inport  Port=2
  Constant : Constant  Value=0
  IsInf : RelationalOperator  Operator=isInf  OutDataTypeStr=boolean  RndMeth=Simplest  InputSameDT=off
  IsNaN : RelationalOperator  Operator=isNaN  OutDataTypeStr=boolean  RndMeth=Simplest  InputSameDT=off
  Logical Operator : Logic  Operator=OR  Inputs=3  AllPortsSameDT=off  OutDataTypeStr=boolean
  Switch : Switch  Criteria=u2 > Threshold  SaturateOnIntegerOverflow=off  InputSameDT=off
  "I_L_rms_1 " : Outport
  wires:
  Failed?/1 -> Logical Operator/1
  Constant/1 -> Switch/1
  I_L_rms_1/1 -> IsNaN/1, IsInf/1, Switch/3
  Switch/1 -> "I_L_rms_1 "/1
  Logical Operator/1 -> Switch/2
  IsNaN/1 -> Logical Operator/2
  IsInf/1 -> Logical Operator/3

== system Lib_EMTAT/Components/Power Flow/AC-AC Transformer (Power Loss Map)/Open Circuit Failure - Line to Neutral Voltage ==
  Failed? : Inport
  V_LN_rms_2 : Inport  Port=2
  Constant : Constant  Value=0
  IsInf : RelationalOperator  Operator=isInf  OutDataTypeStr=boolean  RndMeth=Simplest  InputSameDT=off
  IsNaN : RelationalOperator  Operator=isNaN  OutDataTypeStr=boolean  RndMeth=Simplest  InputSameDT=off
  Logical Operator : Logic  Operator=OR  Inputs=3  AllPortsSameDT=off  OutDataTypeStr=boolean
  Switch : Switch  Criteria=u2 > Threshold  SaturateOnIntegerOverflow=off  InputSameDT=off
  "V_LN_rms_2 " : Outport
  wires:
  IsInf/1 -> Logical Operator/3
  IsNaN/1 -> Logical Operator/2
  Logical Operator/1 -> Switch/2
  Switch/1 -> "V_LN_rms_2 "/1
  V_LN_rms_2/1 -> Switch/3, IsInf/1, IsNaN/1
  Constant/1 -> Switch/1
  Failed?/1 -> Logical Operator/1

== system Lib_EMTAT/Components/Power Flow/AC-AC Transformer (Power Loss Map)/Open Circuit// Degradation Failure ==
  Ploss : Inport
  DegFail? : Inport  Port=2
  OCFail? : Inport  Port=3
  Deg : Inport  Port=4
  Constant : Constant  Value=0
  Constant1 : Constant  Value=Plosslim
  Divide : Product  Inputs=**
  "If degradation failure, add to Ploss." : Switch  Criteria=u2 > Threshold  SaturateOnIntegerOverflow=off  InputSameDT=off
  "If open circuit failure, set Ploss = 0." : Switch  Criteria=u2 > Threshold  SaturateOnIntegerOverflow=off  InputSameDT=off
  Sum1 : Sum  Inputs=++|
  "Ploss " : Outport
  wires:
  DegFail?/1 -> "If degradation failure, add to Ploss."/2
  "If degradation failure, add to Ploss."/1 -> "If open circuit failure, set Ploss = 0."/3
  Ploss/1 -> Sum1/2, "If degradation failure, add to Ploss."/3
  Sum1/1 -> "If degradation failure, add to Ploss."/1
  Deg/1 -> Divide/2
  "If open circuit failure, set Ploss = 0."/1 -> "Ploss "/1
  OCFail?/1 -> "If open circuit failure, set Ploss = 0."/2
  Constant/1 -> "If open circuit failure, set Ploss = 0."/1
  Constant1/1 -> Divide/1
  Divide/1 -> Sum1/1

== system Lib_EMTAT/Components/Power Flow/AC-AC Transformer (Power Loss Map)/Power Loss ==
  V_LN_rms_1 : Inport
  I_L_rms_2 : Inport  Port=2
  2-D Lookup Table : Lookup_n-D  BreakpointsForDimension1=X_C_VoltageAC1Vec_M  BreakpointsForDimension2=Y_C_CurrentAC2Vec_M  Table=T_C_PowLossArray_M  ExtrapMethod=Clip  UseLastTableValue=on  InternalRulePriority=Speed  RndMeth=Simplest
      settings: InputPortMap=u0,u1
  Abs : Abs  SaturateOnIntegerOverflow=off
  Abs1 : Abs  SaturateOnIntegerOverflow=off
  Saturation : Saturate  UpperLimit=inf  LowerLimit=0
  Ploss : Outport
  wires:
  V_LN_rms_1/1 -> Abs/1
  Abs/1 -> 2-D Lookup Table/1
  Abs1/1 -> 2-D Lookup Table/2
  I_L_rms_2/1 -> Abs1/1
  2-D Lookup Table/1 -> Saturation/1
  Saturation/1 -> Ploss/1

== system Lib_EMTAT/Components/Power Flow/AC-DC Rectifier (Efficiency Map)/Compensate for Divide By Zero. ==
  note: If Vin is not equal to zero, use its value.
      | If Vin is equal to zero, it will calculate a nan value for Iin. Set Iin to zero.
  PEquivAC : Inport
  V_LN_rms : Inport  Port=2
  Fix Divide By Zero. : Subsystem
  I_L_rms : Outport
  wires:
  V_LN_rms/1 -> Fix Divide By Zero./1(V_LN_rms)
  PEquivAC/1 -> Fix Divide By Zero./2(PEquivAC)
  Fix Divide By Zero./1(I_L_rms) -> I_L_rms/1

== system Lib_EMTAT/Components/Power Flow/AC-DC Rectifier (Efficiency Map)/Direction Determination ==
  P_DC : Inport
  Eff : Inport  Port=2
  Divide : Product  Inputs=**
  Divide1 : Product  Inputs=*/
  Switch : Switch  Criteria=u2 > Threshold  SaturateOnIntegerOverflow=off  InputSameDT=off
  PEquivAC : Outport
  wires:
  P_DC/1 -> Divide1/1, Divide/2, Switch/2
  Divide/1 -> Switch/1
  Divide1/1 -> Switch/3
  Eff/1 -> Divide/1, Divide1/2
  Switch/1 -> PEquivAC/1

== system Lib_EMTAT/Components/Power Flow/AC-DC Rectifier (Efficiency Map)/Efficiency ==
  V_DC : Inport
  I_L_rms : Inport  Port=2
  2-D Lookup Table : Lookup_n-D  BreakpointsForDimension1=X_C_VoltageInVec_M  BreakpointsForDimension2=Y_C_RMSCurrentOutVec_M  Table=T_C_EffArray_M  ExtrapMethod=Clip  UseLastTableValue=on  InternalRulePriority=Speed  RndMeth=Simplest
      settings: InputPortMap=u0,u1
  Abs : Abs  SaturateOnIntegerOverflow=off
  Abs1 : Abs  SaturateOnIntegerOverflow=off
  Eff : Outport
  wires:
  2-D Lookup Table/1 -> Eff/1
  I_L_rms/1 -> Abs1/1
  Abs1/1 -> 2-D Lookup Table/2
  Abs/1 -> 2-D Lookup Table/1
  V_DC/1 -> Abs/1

== system Lib_EMTAT/Components/Power Flow/AC-DC Rectifier (Efficiency Map)/Failure Determination ==
  Fail? : Inport
  Compare To Constant : simulink/Logic and Bit Operations/Compare To Constant  relop===  const=1  OutDataTypeStr=boolean
  Compare To Constant1 : simulink/Logic and Bit Operations/Compare To Constant  relop===  const=2  OutDataTypeStr=boolean
  Data Type Conversion : DataTypeConversion  OutDataTypeStr=double  SaturateOnIntegerOverflow=off  RndMeth=Floor
  Data Type Conversion1 : DataTypeConversion  OutDataTypeStr=double  SaturateOnIntegerOverflow=off  RndMeth=Floor
  Failure Mode : Constant  Value=FM
  Logical Operator : Logic  AllPortsSameDT=off  OutDataTypeStr=boolean
  Logical Operator1 : Logic  AllPortsSameDT=off  OutDataTypeStr=boolean
  OCFail : Outport
  DegFail : Outport  Port=2
  wires:
  Data Type Conversion/1 -> OCFail/1
  Data Type Conversion1/1 -> DegFail/1
  Fail?/1 -> Logical Operator/2, Logical Operator1/2
  Logical Operator1/1 -> Data Type Conversion1/1
  Compare To Constant1/1 -> Logical Operator1/1
  Logical Operator/1 -> Data Type Conversion/1
  Compare To Constant/1 -> Logical Operator/1
  Failure Mode/1 -> Compare To Constant/1, Compare To Constant1/1

== system Lib_EMTAT/Components/Power Flow/AC-DC Rectifier (Efficiency Map)/Open Circuit Failure - DC Voltage ==
  Failed? : Inport
  V_DC : Inport  Port=2
  Constant : Constant  Value=0
  IsInf : RelationalOperator  Operator=isInf  OutDataTypeStr=boolean  RndMeth=Simplest  InputSameDT=off
  IsNaN : RelationalOperator  Operator=isNaN  OutDataTypeStr=boolean  RndMeth=Simplest  InputSameDT=off
  Logical Operator : Logic  Operator=OR  Inputs=3  AllPortsSameDT=off  OutDataTypeStr=boolean
  Switch : Switch  Criteria=u2 > Threshold  SaturateOnIntegerOverflow=off  InputSameDT=off
  "V_DC " : Outport
  wires:
  IsInf/1 -> Logical Operator/3
  IsNaN/1 -> Logical Operator/2
  Logical Operator/1 -> Switch/2
  Switch/1 -> "V_DC "/1
  V_DC/1 -> Switch/3, IsInf/1, IsNaN/1
  Constant/1 -> Switch/1
  Failed?/1 -> Logical Operator/1
